simulink model "segway_ctrl"  (R2020a)
settings: Solver=daessc  StartTime=0.0  StopTime=simlength  MaxStep=ts  RelTol=1e-3
values from neighbouring files (symbols this model uses):
  A = [a11 a12 a13 a14; a21 a22 a23 a24; a31 a32 a33 a34; a41 a42 a43 a44]    [init_segway_ctrl.m]
  B = [0 b2 0 b4]'    [init_segway_ctrl.m]
  C = [1 0 0 0; 0 0 1 0]    [init_segway_ctrl.m]
  g = 9.8    [init_segway_ctrl.m]
  Ke1 = acker(Ae,Be,poles_sf)    [init_segway_ctrl.m]
  L = (place(A',C',poles_obs))'    [init_segway_ctrl.m]
  omega_1_ref = vref/r1    (= 28.5714285714)    [init_segway_ctrl.m]
  simlength = 20    [init_segway_ctrl.m]
libraries: nesl_utility x7, simulink x1, segway_lib x1
settings Model: SimulationMode=accelerator  Creator=dbagn  LastModifiedBy=dabagnara
settings DataIOCC: ReturnWorkspaceOutputs=off

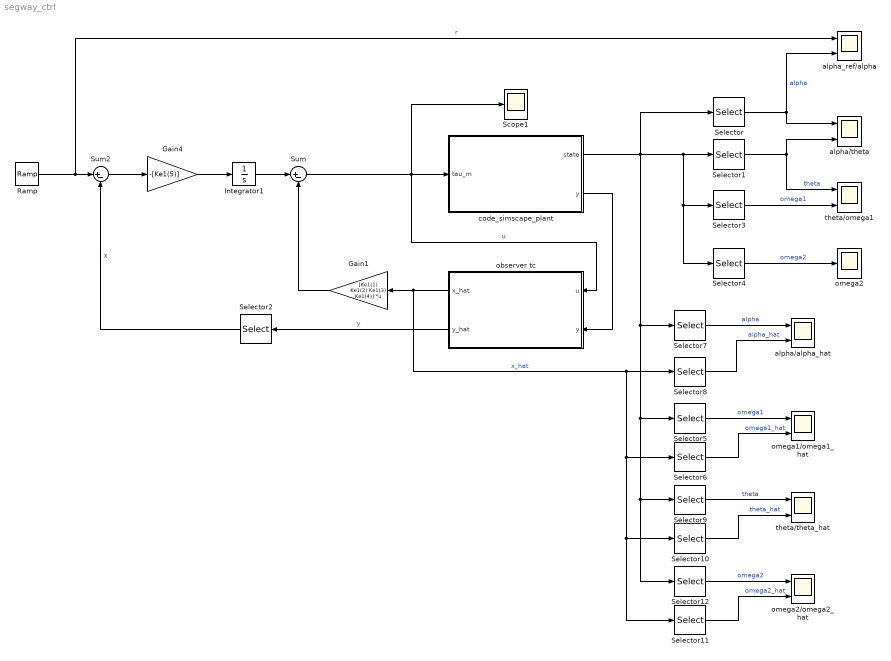
== system segway_ctrl ==
  Gain1 : Gain  Gain=[Ke1(1) Ke1(2) Ke1(3) Ke1(4)]  Multiplication=Matrix(K*u)
  Gain4 : Gain  Gain=-[Ke1(5)]
  Integrator1 : Integrator
  Ramp : simulink/Sources/Ramp  slope=omega_1_ref  start=0  InitialOutput=0
  Scope1 : Scope
  Selector : Selector  InputPortWidth=4  IndexOptions=Index vector (dialog)  Indices=1  OutputSizes=1
  Selector1 : Selector  InputPortWidth=4  IndexOptions=Index vector (dialog)  Indices=3  OutputSizes=1
  Selector10 : Selector  InputPortWidth=4  IndexOptions=Index vector (dialog)  Indices=3  OutputSizes=1
  Selector11 : Selector  InputPortWidth=4  IndexOptions=Index vector (dialog)  Indices=4  OutputSizes=1
  Selector12 : Selector  InputPortWidth=4  IndexOptions=Index vector (dialog)  Indices=4  OutputSizes=1
  Selector2 : Selector  InputPortWidth=2  IndexOptions=Index vector (dialog)  Indices=1  OutputSizes=1
  Selector3 : Selector  InputPortWidth=4  IndexOptions=Index vector (dialog)  Indices=2  OutputSizes=1
  Selector4 : Selector  InputPortWidth=4  IndexOptions=Index vector (dialog)  Indices=4  OutputSizes=1
  Selector5 : Selector  InputPortWidth=4  IndexOptions=Index vector (dialog)  Indices=2  OutputSizes=1
  Selector6 : Selector  InputPortWidth=4  IndexOptions=Index vector (dialog)  Indices=2  OutputSizes=1
  Selector7 : Selector  InputPortWidth=4  IndexOptions=Index vector (dialog)  Indices=1  OutputSizes=1
  Selector8 : Selector  InputPortWidth=4  IndexOptions=Index vector (dialog)  Indices=1  OutputSizes=1
  Selector9 : Selector  InputPortWidth=4  IndexOptions=Index vector (dialog)  Indices=3  OutputSizes=1
  Sum : Sum  Inputs=|+-
  Sum2 : Sum  Inputs=|+-
  alpha/alpha_hat : Scope  NumInputPorts=2
  alpha/theta : Scope  NumInputPorts=2
  alpha_ref/alpha : Scope  NumInputPorts=2
  "code_simscape_plant " : Subsystem
  observer tc : Subsystem
  omega1/omega1_hat : Scope  NumInputPorts=2
  omega2 : Scope
  omega2/omega2_hat : Scope  NumInputPorts=2
  theta/omega1 : Scope  NumInputPorts=2
  theta/theta_hat : Scope  NumInputPorts=2
  wires:
  Selector/1 -> alpha/theta/1, alpha_ref/alpha/2  "alpha"
  "code_simscape_plant "/2(y) -> observer tc/2(y)
  observer tc/2(y_hat) -> Selector2/1  "y"
  Ramp/1 -> alpha_ref/alpha/1, Sum2/1  "r"
  Gain4/1 -> Integrator1/1
  Sum2/1 -> Gain4/1
  Selector1/1 -> theta/omega1/1, alpha/theta/2  "theta"
  "code_simscape_plant "/1(state) -> Selector/1, Selector12/1, Selector9/1, Selector5/1, Selector7/1, Selector4/1, Selector3/1, Selector1/1
  Gain1/1 -> Sum/2
  observer tc/1(x_hat) -> Selector8/1, Selector11/1, Selector10/1, Selector6/1, Gain1/1  "x_hat"
  Selector2/1 -> Sum2/2  "x"
  Sum/1 -> Scope1/1, "code_simscape_plant "/1(tau_m), observer tc/1(u)  "u"
  Selector3/1 -> theta/omega1/2  "omega1"
  Selector4/1 -> omega2/1  "omega2"
  Integrator1/1 -> Sum/1
  Selector5/1 -> omega1/omega1_hat/1  "omega1"
  Selector6/1 -> omega1/omega1_hat/2  "omega1_hat"
  Selector7/1 -> alpha/alpha_hat/1  "alpha"
  Selector8/1 -> alpha/alpha_hat/2  "alpha_hat"
  Selector10/1 -> theta/theta_hat/2  "theta_hat"
  Selector9/1 -> theta/theta_hat/1  "theta"
  Selector12/1 -> omega2/omega2_hat/1  "omega2"
  Selector11/1 -> omega2/omega2_hat/2  "omega2_hat"

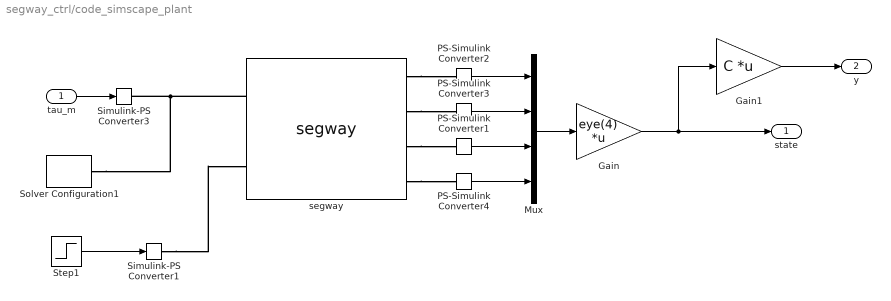
== system segway_ctrl/code_simscape_plant  ==
  tau_m : Inport
  Gain : Gain  Gain=eye(4)  Multiplication=Matrix(K*u)
  Gain1 : Gain  Gain=C  Multiplication=Matrix(K*u)
  Mux : Mux
  PS-Simulink Converter1 : nesl_utility/PS-Simulink Converter  PhysicalDomain=network_engine_domain  SubClassName=ps_output  LeftPortType=input  RightPortType=output  PseudoPeriodic=off  Frequencies=[]  Unit=rad  AffineConversion=on
  PS-Simulink Converter2 : nesl_utility/PS-Simulink Converter  PhysicalDomain=network_engine_domain  SubClassName=ps_output  LeftPortType=input  RightPortType=output  PseudoPeriodic=off  Frequencies=[]  Unit=rad  AffineConversion=on
  PS-Simulink Converter3 : nesl_utility/PS-Simulink Converter  PhysicalDomain=network_engine_domain  SubClassName=ps_output  LeftPortType=input  RightPortType=output  PseudoPeriodic=off  Frequencies=[]  Unit=rad/s  AffineConversion=on
  PS-Simulink Converter4 : nesl_utility/PS-Simulink Converter  PhysicalDomain=network_engine_domain  SubClassName=ps_output  LeftPortType=input  RightPortType=output  PseudoPeriodic=off  Frequencies=[]  Unit=rad/s  AffineConversion=on
  Simulink-PS Converter1 : nesl_utility/Simulink-PS Converter  PhysicalDomain=network_engine_domain  SubClassName=ps_input  LeftPortType=input  RightPortType=output  PseudoPeriodic=off  Frequencies=[]  NoiseDistribution=none  NoiseParameters=[]  Unit=N*m  AffineConversion=off  FilteringAndDerivatives=provide  SimscapeFilterOrder=1  InputFilterTimeConstant=0.001  UdotUserProvided=0
  Simulink-PS Converter3 : nesl_utility/Simulink-PS Converter  PhysicalDomain=network_engine_domain  SubClassName=ps_input  LeftPortType=input  RightPortType=output  PseudoPeriodic=off  Frequencies=[]  NoiseDistribution=none  NoiseParameters=[]  Unit=N*m  AffineConversion=off  FilteringAndDerivatives=provide  SimscapeFilterOrder=1  InputFilterTimeConstant=0.001  UdotUserProvided=0
  Solver Configuration1 : nesl_utility/Solver Configuration  PhysicalDomain=network_engine_domain  SubClassName=solver  LeftPortType=input  RightPortType=generic  Tones=[]  Harmonics=[]  SimulateNoise=off  Profile=off  UseLocalSampling=off  EnableSwitchedLinearOptims=on  FrequencyDomain=off  UseCCode=off  RelTol=0.001  AbsTol=1e-06  MinStep=1e-09  ToWorkspace=off  RevertToSquareIcSolve=off  NumHomotopyIterations=100  PhasorMode=off  PhasorModeNumHarmonics=1  DoDC=on  ResidualTolerance=1e-09  UseLocalSolver=on  LocalSolverChoice=NE_BACKWARD_EULER_ADVANCER  LocalSolverSampleTime=ts  DoFixedCost=on  MaxNonlinIter=3  MaxModeIter=2  LinearAlgebra=auto  EquationFormulation=NE_TIME_EF  DelaysMemoryBudget=1024  AutomaticFiltering=on  FilteringTimeConstant=0.001  PartitionStorageMethod=AS_NEEDED  PartitionMemoryBudget=1024  PartitionMethod=ROBUST
  Step1 : Step  Time=simlength/2  After=250  SampleTime=0
  segway : segway_lib/segway  m1=m1 kg  m2=m2 kg  J1=J1 kg*m^2  J2=J2 kg*m^2  r1=r1 m  r2=r2 m  b1=b1 N*m/(rad/s)  b2=b2 N*m/(rad/s)  g=g m/s^2  x1_specify=off  x1_priority=None  x1=0 rad  x1_nominal_specify=off  x1_nominal_unit=rad  x1_nominal_value=1  x2_specify=off  x2_priority=None  x2=0 rad/s  x2_nominal_specify=off  x2_nominal_unit=rad/s  x2_nominal_value=1  x3_specify=on  x3_priority=High  x3=1 rad  x3_nominal_specify=off  x3_nominal_unit=rad  x3_nominal_value=1  x4_specify=on  x4_priority=High  x4=0 rad/s  x4_nominal_specify=off  x4_nominal_unit=rad/s  x4_nominal_value=1
      settings: InternalSimscapePortConfiguration="{\"Bottom\":[],\"Left\":[{\"id\":\"tau_m\",\"label\":\"tau_m\",\"type\":\"input\"},{\"id\":\"d\",\"label\":\"d\",\"type\":\"input\"}],\"Right\":[{\"id\":\"alpha\",\"label\":\"alpha\",\"type\":\"output\"},{\"id\":\"omega_1\",\"label\":\"omega_1\",\"type\":\"output\"},{\"id\":\"theta\",\"label\":\"theta\",\"type\":\"output\"},{\"id\":\"omega_2\",\"label\":\"omega_2\",\"type\":\"output\"}],\"Top\":[]}"
  state : Outport
  y : Outport  Port=2
  wires:
  PS-Simulink Converter2/1 -> Mux/1
  PS-Simulink Converter3/1 -> Mux/2
  tau_m/1 -> Simulink-PS Converter3/1
  PS-Simulink Converter1/1 -> Mux/3
  PS-Simulink Converter4/1 -> Mux/4
  Mux/1 -> Gain/1
  Gain/1 -> Gain1/1, state/1
  Gain1/1 -> y/1
  Step1/1 -> Simulink-PS Converter1/1
  connections:
  segway/RConn4 -- PS-Simulink Converter4/LConn1
  segway/RConn3 -- PS-Simulink Converter1/LConn1
  segway/RConn2 -- PS-Simulink Converter3/LConn1
  segway/RConn1 -- PS-Simulink Converter2/LConn1
  segway/LConn1 -- Solver Configuration1/RConn1 -- Simulink-PS Converter3/RConn1
  Simulink-PS Converter1/RConn1 -- segway/LConn2

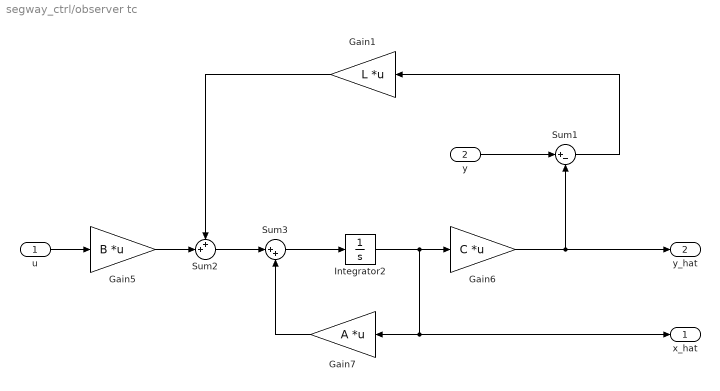
== system segway_ctrl/observer tc ==
  u : Inport
  y : Inport  Port=2
  Gain1 : Gain  Gain=L  Multiplication=Matrix(K*u)
  Gain5 : Gain  Gain=B  Multiplication=Matrix(K*u)
  Gain6 : Gain  Gain=C  Multiplication=Matrix(K*u)
  Gain7 : Gain  Gain=A  Multiplication=Matrix(K*u)
  Integrator2 : Integrator  InitialCondition=[0 0 0 0]
  Sum1 : Sum  Inputs=|+-
  Sum2 : Sum  Inputs=++|
  Sum3 : Sum  Inputs=|++
  x_hat : Outport
  y_hat : Outport  Port=2
  wires:
  Sum2/1 -> Sum3/1
  Integrator2/1 -> x_hat/1, Gain7/1, Gain6/1
  Sum3/1 -> Integrator2/1
  Gain7/1 -> Sum3/2
  y/1 -> Sum1/1
  Gain6/1 -> y_hat/1, Sum1/2
  Sum1/1 -> Gain1/1
  u/1 -> Gain5/1
  Gain1/1 -> Sum2/1
  Gain5/1 -> Sum2/2
